simulink model "moeladod"  (R2018a)
settings: Solver=VariableStepAuto  StartTime=0.0  StopTime=8  RelTol=1e-3
settings Model: Creator=410  LastModifiedBy=410
settings DataIOCC: ReturnWorkspaceOutputs=on
settings SFSimCC: SimUseLocalCustomCode=on
settings RTWCC: RTWUseLocalCustomCode=on

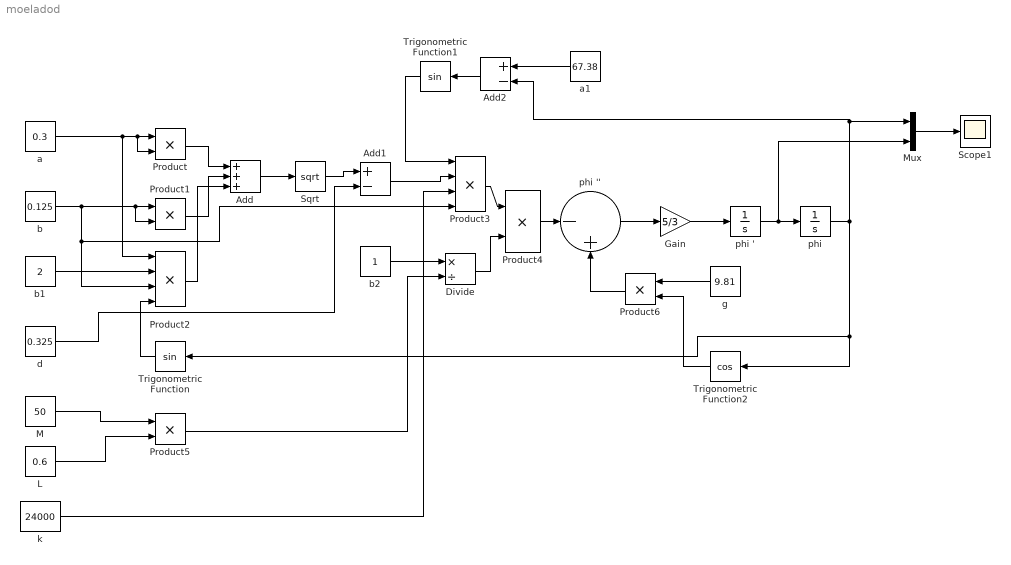
== system moeladod ==
  Add : Sum  Inputs=+++
  Add1 : Sum  Inputs=+-
  Add2 : Sum  Inputs=+-
  Divide : Product  Inputs=*/
  Gain : Gain  Gain=5/3
  "L " : Constant  Value=0.6
  M : Constant  Value=50
  Mux : Mux  Inputs=2
  Product{,1,4..6} (5 alike) : Product
  Product2 : Product  Inputs=4
  Product3 : Product  Inputs=4
  Scope1 : Scope
  Sqrt : Sqrt  SaturateOnIntegerOverflow=on
  Trigonometric Function : Trigonometry
  Trigonometric Function1 : Trigonometry
  Trigonometric Function2 : Trigonometry  Operator=cos
  a : Constant  Value=0.3
  a1 : Constant  Value=67.38
  b : Constant  Value=0.125
  b1 : Constant  Value=2
  b2 : Constant
  d : Constant  Value=0.325
  "g " : Constant  Value=9.81
  "k " : Constant  Value=24000
  phi : Integrator
  phi ' : Integrator
  phi '' : Sum  Inputs=|-+
  wires:
  phi '/1 -> Mux/2, phi/1
  phi ''/1 -> Gain/1
  Gain/1 -> phi '/1
  a/1 -> Product2/1, Product/2, Product/1
  b/1 -> Product2/3, Product3/4, Product1/2, Product1/1
  Product/1 -> Add/1
  Product1/1 -> Add/2
  Add/1 -> Sqrt/1
  phi/1 -> Mux/1, Add2/2, Trigonometric Function2/1, Trigonometric Function/1
  b1/1 -> Product2/2
  Product2/1 -> Add/3
  Sqrt/1 -> Add1/1
  d/1 -> Add1/2
  Add1/1 -> Product3/2
  a1/1 -> Add2/1
  Add2/1 -> Trigonometric Function1/1
  Trigonometric Function1/1 -> Product3/1
  "k "/1 -> Product3/3
  Product3/1 -> Product4/1
  Product4/1 -> phi ''/1
  M/1 -> Product5/1
  "L "/1 -> Product5/2
  Product5/1 -> Divide/2
  b2/1 -> Divide/1
  Divide/1 -> Product4/2
  "g "/1 -> Product6/1
  Trigonometric Function2/1 -> Product6/2
  Product6/1 -> phi ''/2
  Mux/1 -> Scope1/1
  Trigonometric Function/1 -> Product2/4
